simulink model "sys_2D"  (R2019a)
settings: Solver=VariableStepAuto  StartTime=0.0  StopTime=10  FixedStep=0.001  MaxStep=0.01  RelTol=1e-4
undefined symbols (not defined in the file): c, ddxd, ddyd, dx0, dxd, dy0, dyd, frx, fry, k, K1, K2, m, time_scale, x0, xd, y0, yd
settings Model: Creator=程红太  LastModifiedBy=zw
settings DataIOCC: ReturnWorkspaceOutputs=off
settings DebuggingCC: ArithmeticOperatorsInVariantConditions=warning
settings SFSimCC: SimUseLocalCustomCode=off
settings RTWCC: RTWUseLocalCustomCode=off

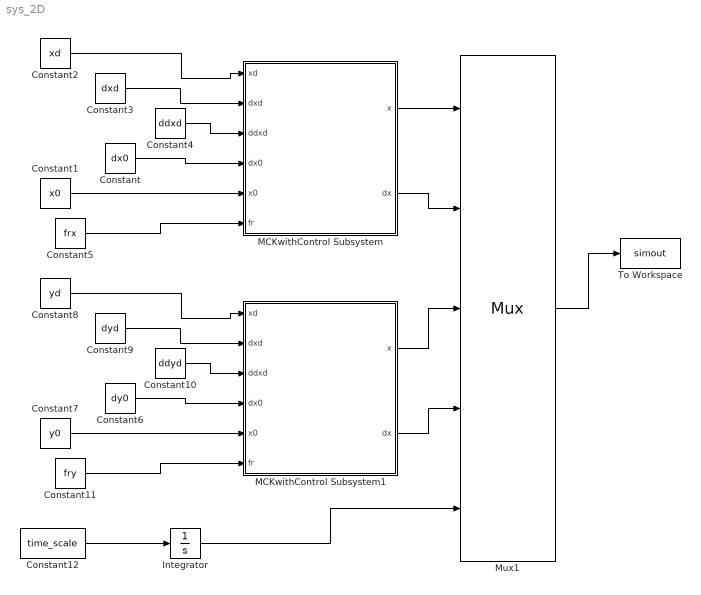
== system sys_2D ==
  Constant : Constant  Value=dx0
  Constant1 : Constant  Value=x0
  Constant10 : Constant  Value=ddyd
  Constant11 : Constant  Value=fry  OutDataTypeStr=double
  Constant12 : Constant  Value=time_scale  OutDataTypeStr=double
  Constant2 : Constant  Value=xd
  Constant3 : Constant  Value=dxd
  Constant4 : Constant  Value=ddxd
  Constant5 : Constant  Value=frx  OutDataTypeStr=double
  Constant6 : Constant  Value=dy0
  Constant7 : Constant  Value=y0
  Constant8 : Constant  Value=yd
  Constant9 : Constant  Value=dyd
  Integrator : Integrator
  MCKwithControl Subsystem : Subsystem
  MCKwithControl Subsystem1 : Subsystem
  Mux1 : Mux  Inputs=5
  To Workspace : ToWorkspace  VariableName=simout  SaveFormat=Structure With Time  SampleTime=-1
  wires:
  Constant/1 -> MCKwithControl Subsystem/4(dx0)
  Constant1/1 -> MCKwithControl Subsystem/5(x0)
  Constant2/1 -> MCKwithControl Subsystem/1(xd)
  Constant3/1 -> MCKwithControl Subsystem/2(dxd)
  Constant4/1 -> MCKwithControl Subsystem/3(ddxd)
  MCKwithControl Subsystem/1(x) -> Mux1/1
  Mux1/1 -> To Workspace/1
  Constant5/1 -> MCKwithControl Subsystem/6(fr)
  MCKwithControl Subsystem/2(dx) -> Mux1/2
  Constant11/1 -> MCKwithControl Subsystem1/6(fr)
  Constant10/1 -> MCKwithControl Subsystem1/3(ddxd)
  Constant9/1 -> MCKwithControl Subsystem1/2(dxd)
  Constant8/1 -> MCKwithControl Subsystem1/1(xd)
  Constant7/1 -> MCKwithControl Subsystem1/5(x0)
  Constant6/1 -> MCKwithControl Subsystem1/4(dx0)
  MCKwithControl Subsystem1/1(x) -> Mux1/3
  MCKwithControl Subsystem1/2(dx) -> Mux1/4
  Integrator/1 -> Mux1/5
  Constant12/1 -> Integrator/1

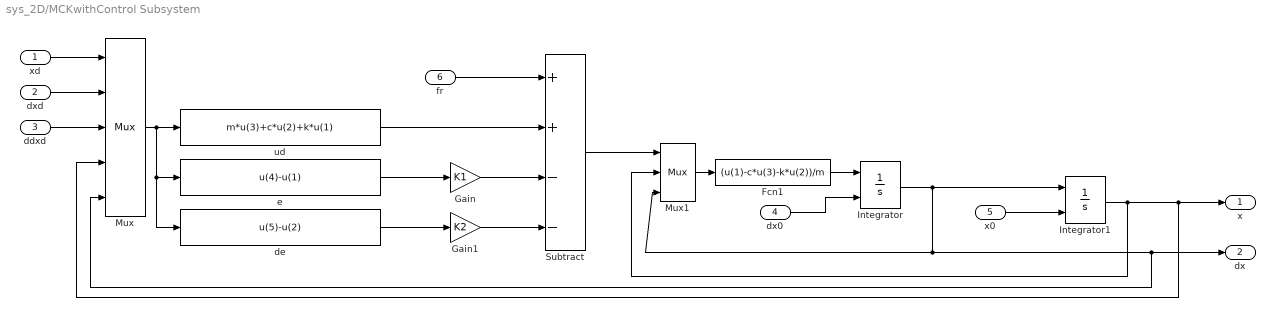
== system sys_2D/MCKwithControl Subsystem ==
  xd : Inport
  dxd : Inport  Port=2
  ddxd : Inport  Port=3
  dx0 : Inport  Port=4
  x0 : Inport  Port=5
  fr : Inport  Port=6
  Fcn1 : Fcn  Expr=(u(1)-c*u(3)-k*u(2))/m
  Gain : Gain  Gain=K1
  Gain1 : Gain  Gain=K2
  Integrator : Integrator  InitialConditionSource=external
  Integrator1 : Integrator  InitialConditionSource=external
  Mux : Mux  Inputs=5
  Mux1 : Mux  Inputs=3
  Subtract : Sum  Inputs=++--
  de : Fcn  Expr=u(5)-u(2)
  e : Fcn  Expr=u(4)-u(1)
  ud : Fcn  Expr=m*u(3)+c*u(2)+k*u(1)
  x : Outport
  dx : Outport  Port=2
  wires:
  dx0/1 -> Integrator/2
  Integrator/1 -> dx/1, Mux/5, Mux1/3, Integrator1/1
  Fcn1/1 -> Integrator/1
  Mux1/1 -> Fcn1/1
  x0/1 -> Integrator1/2
  Integrator1/1 -> x/1, Mux/4, Mux1/2
  ddxd/1 -> Mux/3
  Mux/1 -> de/1, e/1, ud/1
  dxd/1 -> Mux/2
  xd/1 -> Mux/1
  ud/1 -> Subtract/2
  Subtract/1 -> Mux1/1
  fr/1 -> Subtract/1
  e/1 -> Gain/1
  Gain/1 -> Subtract/3
  de/1 -> Gain1/1
  Gain1/1 -> Subtract/4

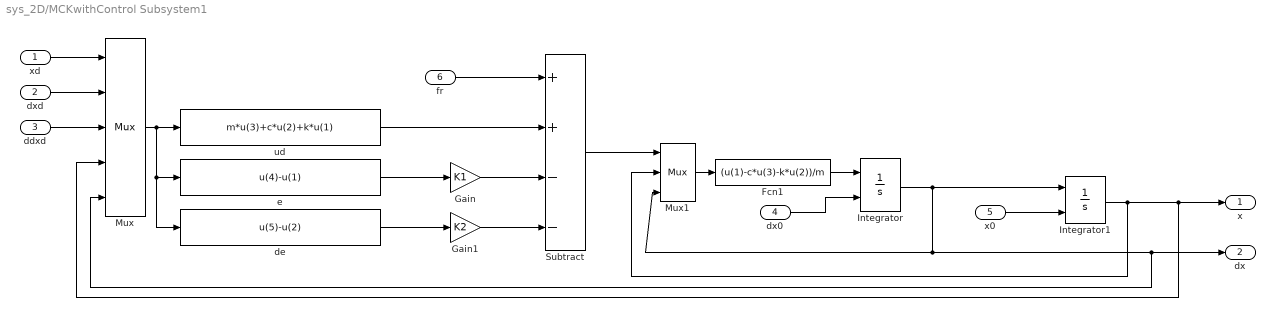
== system sys_2D/MCKwithControl Subsystem1 ==
  xd : Inport
  dxd : Inport  Port=2
  ddxd : Inport  Port=3
  dx0 : Inport  Port=4
  x0 : Inport  Port=5
  fr : Inport  Port=6
  Fcn1 : Fcn  Expr=(u(1)-c*u(3)-k*u(2))/m
  Gain : Gain  Gain=K1
  Gain1 : Gain  Gain=K2
  Integrator : Integrator  InitialConditionSource=external
  Integrator1 : Integrator  InitialConditionSource=external
  Mux : Mux  Inputs=5
  Mux1 : Mux  Inputs=3
  Subtract : Sum  Inputs=++--
  de : Fcn  Expr=u(5)-u(2)
  e : Fcn  Expr=u(4)-u(1)
  ud : Fcn  Expr=m*u(3)+c*u(2)+k*u(1)
  x : Outport
  dx : Outport  Port=2
  wires:
  Gain1/1 -> Subtract/4
  de/1 -> Gain1/1
  Gain/1 -> Subtract/3
  e/1 -> Gain/1
  fr/1 -> Subtract/1
  Subtract/1 -> Mux1/1
  ud/1 -> Subtract/2
  xd/1 -> Mux/1
  dxd/1 -> Mux/2
  Mux/1 -> ud/1, e/1, de/1
  ddxd/1 -> Mux/3
  Integrator1/1 -> Mux1/2, Mux/4, x/1
  x0/1 -> Integrator1/2
  Mux1/1 -> Fcn1/1
  Fcn1/1 -> Integrator/1
  Integrator/1 -> Integrator1/1, Mux1/3, Mux/5, dx/1
  dx0/1 -> Integrator/2
